simulink model "Model_7"  (R2020b)
settings: Solver=VariableStepAuto  StartTime=0.0  StopTime=10.0  RelTol=1e-3
settings Model: Creator=Akarsh  LastModifiedBy=Akarsh

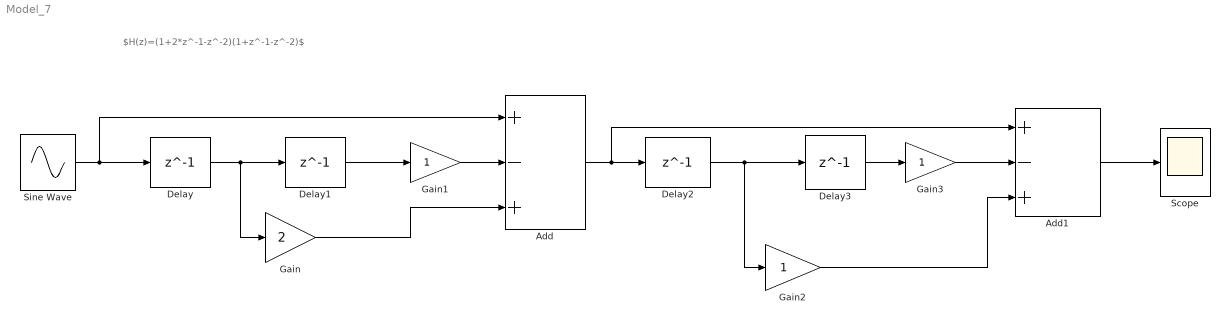
== system Model_7 ==
  note: $H(z)=(1+2*z^-1-z^-2)(1+z^-1-z^-2)$
  Add : Sum  Inputs=+-+
  Add1 : Sum  Inputs=+-+
  Delay{,1..3} (4 alike) : Delay  DelayLength=1
  Gain : Gain  Gain=2
  Gain1 : Gain
  Gain2 : Gain
  Gain3 : Gain
  Scope : Scope
  Sine Wave : Sin  SampleTime=0
  wires:
  Sine Wave/1 -> Add/1, Delay/1
  Delay/1 -> Gain/1, Delay1/1
  Delay1/1 -> Gain1/1
  Gain1/1 -> Add/2
  Gain/1 -> Add/3
  Add/1 -> Add1/1, Delay2/1
  Delay2/1 -> Gain2/1, Delay3/1
  Gain3/1 -> Add1/2
  Gain2/1 -> Add1/3
  Delay3/1 -> Gain3/1
  Add1/1 -> Scope/1
